simulink model "FrameRFModulator"  (R2022b)
settings: Solver=VariableStepAuto  StartTime=0.0  StopTime=10.0  RelTol=1e-3
undefined symbols (not defined in the file): CarrierTs, Dimension, Ts
settings Model: Creator=79327  LastModifiedBy=79327

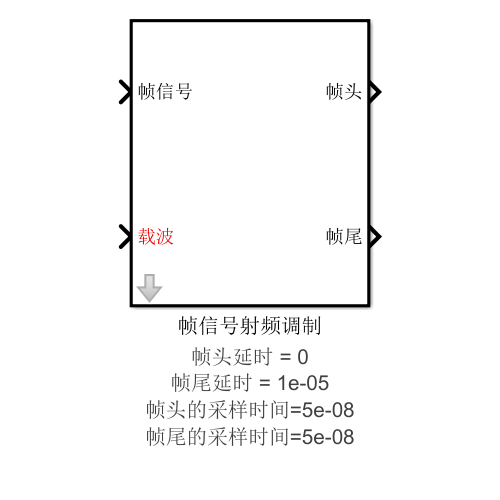
[thumbnail: Simulink's stored preview of the top-level diagram]
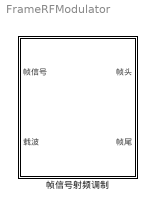
== system FrameRFModulator ==
  帧信号射频调制 : Subsystem  TreatAsAtomicUnit=on  mask{Gain1=0.4, Gain2=0.714, Delay=1e-5, Delay_frameheader=0, Delay_frameend=1e-05, T_frameheader=5e-08, T_frameend=5e-08, CarrierTs=CarrierTs}
      mask prompts: Gain1 "部分载波相乘的增益"; Gain2 "射频调制信号的增益"; Delay "帧头与帧尾之间的延时(s)"; Delay_frameheader "帧头信号的时延"; Delay_frameend "帧尾信号的时延"; T_frameheader "帧头的采样时间"; T_frameend "帧尾的采样时间"; CarrierTs "载波采样时间"
      mask init:
      | %获得模块的句柄
      |             modelpath = gcb;
      |             model = getSimulinkBlockHandle(modelpath,true);
      |             modelDelay = str2double(get_param(model,'Delay'));
      | 
      |             %设置帧头延时
      |             set_param(model,'Delay_frameheader',num2str(0))
      |             %设置帧尾延时
      |             set_param(model,'Delay_frameend',num2str(modelDelay))
      |             %设置帧头信号的采样时间
      |             set_param(model,'T_frameheader',num2str(CarrierTs));
      |             %设置帧尾信号的采样时间
      |             set_param(model,'T_frameend',num2str(CarrierTs));
      settings: AttributesFormatString=|
      | 帧头延时 = %<Delay_frameheader>
      | 帧尾延时 = %<Delay_frameend>
      | 帧头的采样时间=%<T_frameheader>
      | 帧尾的采样时间=%<T_frameend>
      mask DialogControl ParameterGroupVar Prompt: 参数
      mask DialogControl Container3 Prompt: 输出信号的时延
      mask DialogControl Container4 Prompt: 输出信号的采样时间
      mask DialogControl Container5 Prompt: 全局默认参数

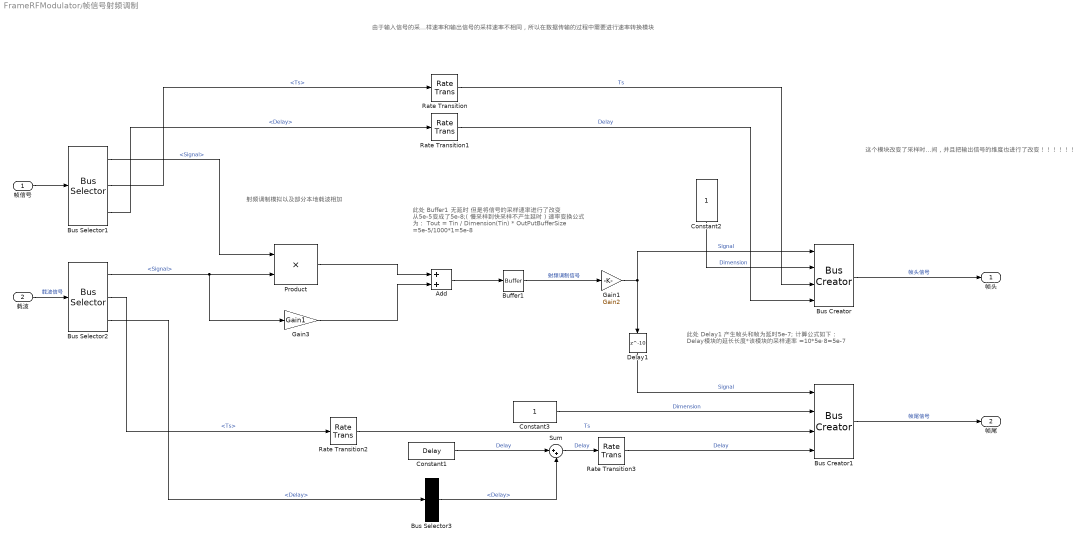
== system FrameRFModulator/帧信号射频调制 ==
  note: 此处 Buffer1 无延时
      | 但是将信号的采样速率进行了改变
      | 从5e-5变成了5e-8;( 慢采样到快采样不产生延时 )
      | 速率变换公式 为：
      | Tout = Tin / Dimension(Tin) * OutPutBufferSize
      | =5e-5/1000*1=5e-8
  note: 射频调制模拟以及部分本地载波相加
  note: 此处 Delay1 产生帧头和帧为延时5e-7;
      | 计算公式如下：
      | Delay模块的延长长度*该模块的采样速率
      | =10*5e·8=5e-7
  note: 由于输入信号的采样速率和输出信号的采样速率不相同，所以在数据传输的过程中需要进行速率转换模块
  note: 这个模块改变了采样时间，并且把输出信号的维度也进行了改变！！！！！！
  帧信号 : Inport  OutDataTypeStr=Bus: SignalBus1
  载波 : Inport  Port=2  OutDataTypeStr=Bus: SignalBus1
  Add : Sum
  Buffer1 : Buffer  N=1  OutputFrames=off
  Bus Creator : BusCreator  Inputs=Signal,Dimension,Ts,Delay  OutDataTypeStr=Bus: SignalBus2  NonVirtualBus=on
  Bus Creator1 : BusCreator  Inputs=Signal,Dimension,Ts,Delay  OutDataTypeStr=Bus: SignalBus2  NonVirtualBus=on
  Bus Selector1 : BusSelector  OutputSignals=Signal,Ts,Delay
  Bus Selector2 : BusSelector  OutputSignals=Signal,Ts,Delay
  Bus Selector3 : BusSelector  OutputSignals=Delay
  Constant1 : Constant  Value=Delay
  Constant2 : Constant
  Constant3 : Constant
  Delay1 : Delay  DelayLength=10  InputProcessing=Columns as channels (frame based)
  Gain1 : Gain  Gain=Gain2
  Gain3 : Gain  Gain=Gain1
  Product : Product
  Rate Transition{,1..3} (4 alike) : RateTransition
  Sum : Sum  Inputs=|++
  帧头 : Outport  OutDataTypeStr=Bus: SignalBus2
  帧尾 : Outport  Port=2  OutDataTypeStr=Bus: SignalBus2
  wires:
  Product/1 -> Add/1
  Gain3/1 -> Add/2
  Add/1 -> Buffer1/1
  Buffer1/1 -> Gain1/1  "射频调制信号"
  Gain1/1 -> Bus Creator/1, Delay1/1  "Signal"
  帧信号/1 -> Bus Selector1/1
  载波/1 -> Bus Selector2/1  "载波信号"
  Bus Creator1/1 -> 帧尾/1  "帧尾信号"
  Bus Creator/1 -> 帧头/1  "帧头信号"
  Delay1/1 -> Bus Creator1/1  "Signal"
  Bus Selector1/1 -> Product/1  "<Signal>"
  Bus Selector2/1 -> Gain3/1, Product/2  "<Signal>"
  Constant1/1 -> Sum/1  "Delay"
  Bus Selector3/1 -> Sum/2  "<Delay>"
  Sum/1 -> Rate Transition3/1  "Delay"
  Bus Selector1/2 -> Rate Transition/1  "<Ts>"
  Constant2/1 -> Bus Creator/2  "Dimension"
  Bus Selector2/2 -> Rate Transition2/1  "<Ts>"
  Bus Selector2/3 -> Bus Selector3/1  "<Delay>"
  Constant3/1 -> Bus Creator1/2  "Dimension"
  Bus Selector1/3 -> Rate Transition1/1  "<Delay>"
  Rate Transition3/1 -> Bus Creator1/4  "Delay"
  Rate Transition2/1 -> Bus Creator1/3  "Ts"
  Rate Transition/1 -> Bus Creator/3  "Ts"
  Rate Transition1/1 -> Bus Creator/4  "Delay"
